simulink model "Optitrack_Simulink_TrackableLocation"  (R2014a)
settings: Solver=ode5  StartTime=0.0  StopTime=inf  FixedStep=0.02  RelTol=1e-3
libraries: rtwinlib x1
settings Model: Creator=sasson  LastModifiedBy=sasson
settings HardwareCC: ProdIntDivRoundTo=Zero  ProdEndianess=LittleEndian  ProdHWDeviceType=Generic->32-bit x86 compatible
settings RTWCC: SystemTargetFile=rtwin.tlc  TemplateMakefile=rtwin.tmf  Description=Real-Time Windows Target  ProcessScript=rtwin_make_rtw_hook  TargetLang=C++  RTWCompilerOptimization=On
settings CodeAppCC: MaxIdLength=95
settings RTWinTargetCC: TargetLibSuffix=_rtwin.lib  TargetPreCompLibLocation=C:\Program Files\MATLAB\R2014a\toolbox\rtw\targets\rtwin\lib\win64

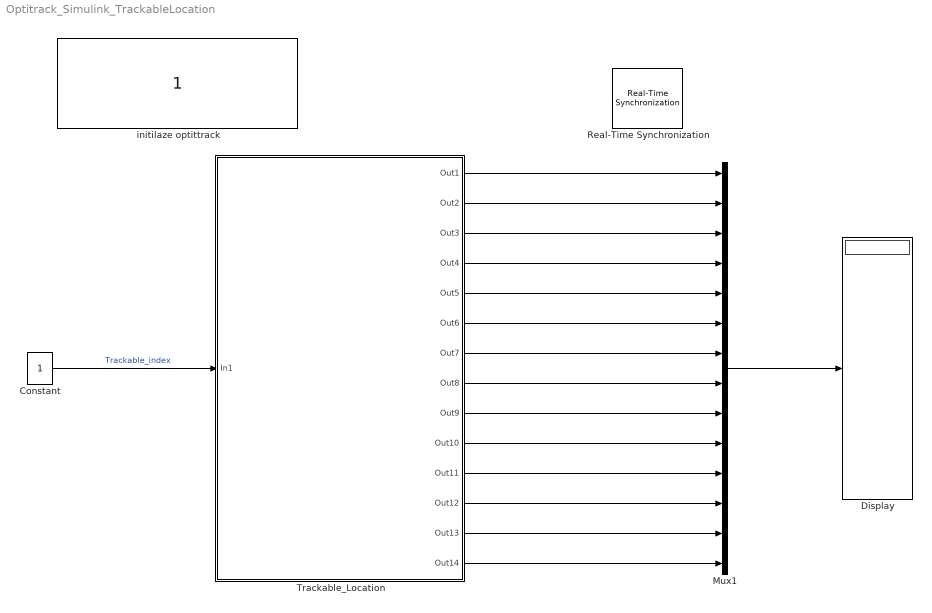
== system Optitrack_Simulink_TrackableLocation ==
  Constant : Constant  OutDataTypeStr=Inherit: Inherit via back propagation
  Display : Display
  Mux1 : Mux  Inputs=14
  Real-Time Synchronization : rtwinlib/Real-Time Synchronization  SampleTime=0.02  MaxMissedTicks=200  ShowMissedTicks=off  YieldWhenWaiting=off
  Trackable_Location : Subsystem
      mask Display:
      | image('optitrack_Trackable.jpg')
      | bgColor = Simulink.Root.ColorString2Rgb(get_param(gcbh, 'BackgroundColor'));
      | disp([10 10 'TrackableLocation']);
      | port_label('output',1,'x');
      | port_label('output',2,'y');
      | port_label('output',3,'z');
      | port_label('output',4,'yaw');
      | port_label('output',5,'pitch');
      | port_label('output',6,'roll');
      | port_label('output',7,'time stamp');
      | port_label('output',8,'Delta Time');
      | port_label('output',9,'dx/dt');
      | port_label('output',10,'dy/dt');
      | port_label('output',11,'dz/dt');
      | port_label('output',12,'dYaw/dt');
      | port_label('output',13,'dPitch/dt');
      | port_label('output',14,'dRoll/dt');
      | 
      | port_label('input',1,'Trackable ID');
  initilaze optittrack : Constant  StartFcn=|  StopFcn=|
      StartFcn=|
      | if ~exist('inc_location')
      |   inc_location =[pwd '\inc']; % change if necessary
      | end
      | 
      | if ~exist('lib_location')
      |   lib_location =[pwd '\inc']; % change if necessary
      | end
      | 
      | % load the NPTrackingTools library if it is not already loaded
      | if ~libisloaded('NPTrackingTools')
      | 
      |     addpath(inc_location); % change if necessary
      |     addpath(lib_location); % change if necessary
      | 
      |    [notfound,warnings]=loadlibrary('NPTrackingToolsx64','NPTrackingTools.h','alias','NPTrackingTools')
      | end
      | 
      | % to see all function write the code: libfunctionsview NPTrackingTools
      | 
      | % initilzing
      | 
      | % libfunctionsview NPTrackingTools --> use this to see available functions
      | 
      | % initialise cameras
      | calllib('NPTrackingTools', 'TT_Initialize') %you should see red leds on the camera turns on
      | %
      | % load the project file which sets up cameras correctly
      | T_old=0;
      | 
      | if ~exist('project_file')
      |    project_file =[pwd '\Motive_1_5_Project.ttp']; % change if necessary
      | end
      | 
      | 
      | calllib('NPTrackingTools', 'TT_LoadProject', project_file)
      StopFcn=|
      | calllib('NPTrackingTools', 'TT_Shutdown') % exit tracking tools
      | unloadlibrary NPTrackingTools
      mask Display:
      | image('optitrack_logo.jpg')
      | color('green');port_label('output',1,'no need to connect')
  wires:
  Constant/1 -> Trackable_Location/1(In1)  "Trackable_index"
  Trackable_Location/1(Out1) -> Mux1/1
  Trackable_Location/2(Out2) -> Mux1/2
  Trackable_Location/3(Out3) -> Mux1/3
  Trackable_Location/4(Out4) -> Mux1/4
  Trackable_Location/5(Out5) -> Mux1/5
  Trackable_Location/6(Out6) -> Mux1/6
  Trackable_Location/7(Out7) -> Mux1/7
  Trackable_Location/8(Out8) -> Mux1/8
  Trackable_Location/9(Out9) -> Mux1/9
  Trackable_Location/10(Out10) -> Mux1/10
  Trackable_Location/11(Out11) -> Mux1/11
  Trackable_Location/12(Out12) -> Mux1/12
  Trackable_Location/13(Out13) -> Mux1/13
  Trackable_Location/14(Out14) -> Mux1/14
  Mux1/1 -> Display/1

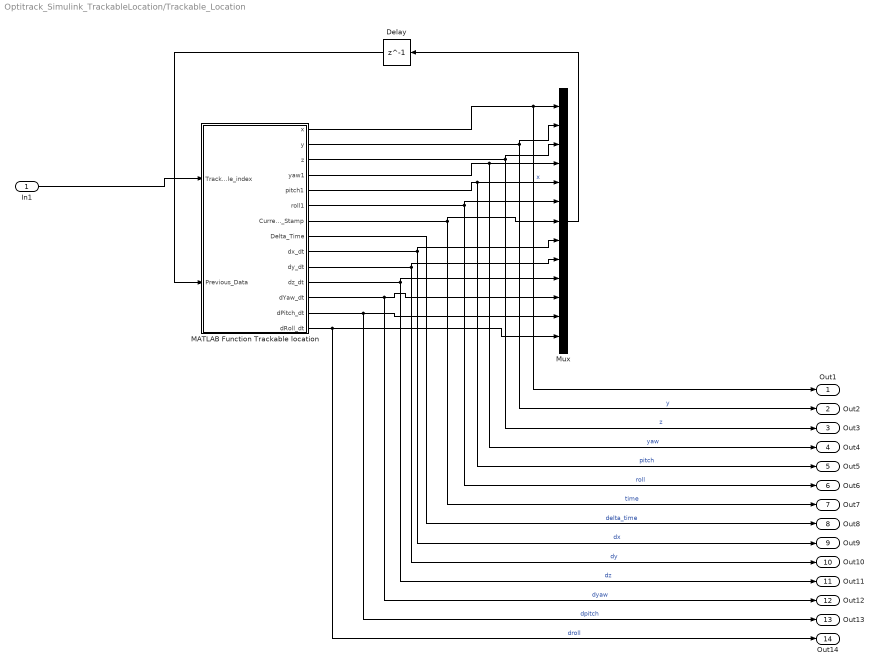
== system Optitrack_Simulink_TrackableLocation/Trackable_Location ==
  In1 : Inport
  Delay : Delay  DelayLength=1  InitialCondition=0
  MATLAB Function Trackable location : MATLAB Function  TreatAsAtomicUnit=on
  Mux : Mux  Inputs=13
  Out1 : Outport
  Out2 : Outport  Port=2
  Out3 : Outport  Port=3
  Out4 : Outport  Port=4
  Out5 : Outport  Port=5
  Out6 : Outport  Port=6
  Out7 : Outport  Port=7
  Out8 : Outport  Port=8
  Out9 : Outport  Port=9
  Out10 : Outport  Port=10
  Out11 : Outport  Port=11
  Out12 : Outport  Port=12
  Out13 : Outport  Port=13
  Out14 : Outport  Port=14
  wires:
  MATLAB Function Trackable location/8(Delta_Time) -> Out8/1  "delta_time"
  MATLAB Function Trackable location/14(dRoll_dt) -> Out14/1, Mux/13  "droll"
  MATLAB Function Trackable location/13(dPitch_dt) -> Out13/1, Mux/12  "dpitch"
  MATLAB Function Trackable location/9(dx_dt) -> Out9/1, Mux/8  "dx"
  MATLAB Function Trackable location/10(dy_dt) -> Out10/1, Mux/9  "dy"
  MATLAB Function Trackable location/11(dz_dt) -> Out11/1, Mux/10  "dz"
  MATLAB Function Trackable location/12(dYaw_dt) -> Mux/11, Out12/1  "dyaw"
  In1/1 -> MATLAB Function Trackable location/1(Trackable_index)
  Mux/1 -> Delay/1
  MATLAB Function Trackable location/6(roll1) -> Out6/1, Mux/6  "roll"
  MATLAB Function Trackable location/5(pitch1) -> Out5/1, Mux/5  "pitch"
  MATLAB Function Trackable location/4(yaw1) -> Out4/1, Mux/4  "yaw"
  MATLAB Function Trackable location/3(z) -> Out3/1, Mux/3  "z"
  MATLAB Function Trackable location/2(y) -> Out2/1, Mux/2  "y"
  MATLAB Function Trackable location/1(x) -> Out1/1, Mux/1  "x"
  MATLAB Function Trackable location/7(Current_Time_Stamp) -> Out7/1, Mux/7  "time"
  Delay/1 -> MATLAB Function Trackable location/2(Previous_Data)

== matlab function Optitrack_Simulink_TrackableLocation/Trackable_Location/MATLAB Function Trackable location ==
  data: Trackable_index input; x output; y output; z output; yaw1 output; pitch1 output; roll1 output; Current_Time_Stamp output; Previous_Data input size=13; Delta_Time output; dx_dt output; dy_dt output; dz_dt output; dYaw_dt output; dPitch_dt output; dRoll_dt output
function [x,y,z,yaw1,pitch1,roll1,Current_Time_Stamp,Delta_Time,...
    dx_dt,dy_dt,dz_dt,dYaw_dt,dPitch_dt,dRoll_dt]=...
    TrackableLocation(Trackable_index,Previous_Data)
    
    coder.extrinsic('calllib') % define matlab function in simulink
    
    %update frame
    calllib('NPTrackingTools', 'TT_Update'); %refresh data
   
    %define the outputs types from TT_TrackableLocation function
    %for the function it's need to be single data type
    X=single(0);Y=single(0);Z=single(0);
    yaw=single(0); pitch=single(0); roll=single(0);
    qx=single(0);qy=single(0);qz=single(0);qw=single(0);
    Current_Time_Stamp=double(0);
    
    
    % find the location of any trackable
    [X,Y,Z,qx,qy,qz,qw,yaw,pitch,roll] = calllib('NPTrackingTools', 'TT_TrackableLocation',(Trackable_index-1),X,Y,Z,qx,qy,qz,qw,yaw,pitch,roll);
    
    % Get Time Stamp
    Current_Time_Stamp = calllib('NPTrackingTools', 'TT_FrameTimeStamp');
    
    % Calculate Time Diffrance Between data pulls
    Delta_Time=Current_Time_Stamp-Previous_Data(7);

    
    % simulink accept only double data type
    x=double(X); y=double(Y); z=double(Z);
    yaw1=double(yaw); pitch1=double(pitch); roll1=double(roll);
    
    
    dx_dt=Previous_Data(8);
    dy_dt=Previous_Data(9);
    dz_dt=Previous_Data(10);
    dYaw_dt=Previous_Data(11);
    dPitch_dt=Previous_Data(12);
    dRoll_dt=Previous_Data(13);
    
    if ~(Delta_Time<=0)
        dx_dt=(x-Previous_Data(1))/Delta_Time;
        dy_dt=(y-Previous_Data(2))/Delta_Time;
        dz_dt=(z-Previous_Data(3))/Delta_Time;
        dYaw_dt=(yaw1-Previous_Data(4))/Delta_Time;
        dPitch_dt=(pitch1-Previous_Data(4))/Delta_Time;
        dRoll_dt=(roll1-Previous_Data(4))/Delta_Time;
    end
    
end
